simulink model "Excavator_Mevea_Bucket"  (R2026a)
settings: Solver=ode23t  StopTime=stopTime  FixedStep=1e-5  MaxStep=Ts  AbsTol=1e-3
PostLoadFcn:
  | set_param(bdroot,'IgnoredZcDiagnostic','none');
  | Excavator_Test_Scenario_Select('loadedBucketDigCycle');
  | Excavator_Mevea_params
StartFcn:
  | tStart = tic;
StopFcn:
  | elapsedSimTime = toc(tStart);
  | disp(['Elapsed Sim Time = ' num2str(elapsedSimTime)]);
model workspace: external: MAT-File ExcavatorAssemblyDataStruct.mat (data not in the file)
undefined symbols (not defined in the file or in its folder): AToBRegOrificeVector, AToTOrificeVector, BiPOrificeVector, BoomC, boomHEArea, boomREArea, boomUpMaxQ, boomValve, BToTOrificeVector, BucketC, bucketCloseMaxQ, bucketOpenMaxQ, BucketR, bucketValve, fluids, gravity, LeftBoomR, maxPumpDisp, minPumpDisp, nominalEngineSpeed, P28Assembly, PToAOrificeVector, PToBOrificeVector, pumpCmdNegRateLimit, pumpCmdPosRateLimit, RightBoomR, StickC, stickInMaxQ, stickOutMaxQ, StickR, stickValve, SwingC, swingDisplacement, swingHighSpeedThreshold, swingMaxQ, SwingR, swingSpeedQGain, swingValve, valveCmdNegRateLimit, valveCmdPosRateLimit, X, Y, Z
libraries: fl_lib x89, sm_lib x79, SimscapeFluids_lib x78, nesl_utility x57, simulink_extras x11, Excavator_Parts_Lib x6, SignalEditorBlockLib x1
(part 7 of 7)

== system Excavator_Mevea_Bucket/Excavator/Hydraulics/ValveBlocks/RightValveBlock/Boom Valve ==
  AtoBRegen : SimscapeFluids_lib/Isothermal Liquid/Valves & Orifices/Orifices/Orifice (IL)  orifice_type=foundation.enum.constant_variable.variable  constant_orifice_spec=fluids.isothermal_liquid.valves_orifices.orifices.enum.constant_orifice_spec.area  variable_orifice_spec=fluids.isothermal_liquid.valves_orifices.orifices.enum.orifice_spec.table1D_area_opening  orifice_area_constant=1e-3 m^2  p_diff_TLU_constant=[-4, -3, -2, -1, -.5, 0, .5, 1, 2, 3, 4] MPa  vol_flow_TLU_constant=[-2.44, -2.12, -1.68, -1.22, -.84, 0, .85, 1.21, 1.7, 2.09, 2.41] .* 1e-3 m^3/s  S_min=1e-10 m  del_S=0.005 m  open_orientation=fluids.isothermal_liquid.valves_orifices.orifices.enum.orifice_orientation.positive  area_max=0.5e-4 m^2  area_leak=1e-12 m^2  S_TLU=valveData.spoolPosVector mm  orifice_area_TLU=valveData.AtoBRegOrificeAreaVector mm^2  area=inf m^2  Cd=0.7  Re_c=150  smoothing_factor=0  pressure_recovery=simscape.enum.onoff.off  S_vol_flow_TLU=AToBRegOrificeVector - 1000*(0) mm  p_diff_TLU=[-10000000, -5000000, -2000000, 2000000, 5000000, 10000000] Pa  vol_flow_TLU=[-1e-07, -7.0711e-08, -4.4721e-08, 4.4721e-08, 7.0711e-08, 1e-07; -2.0352e-05, -1.4391e-05, -9.1017e-06, 9.1017e-06, 1.4391e-05, 2.0352e-05; -.0040736, -.0028805, -.0018218, .0018218, .0028805, .0040736; -.011438, -.0080879, -.0051152, .0051152, .0080879, .011438; -.034356, -.024293, -.015364, .015364, .024293, .034356] m^3/s
  AtoT : SimscapeFluids_lib/Isothermal Liquid/Valves & Orifices/Orifices/Orifice (IL)  orifice_type=foundation.enum.constant_variable.variable  constant_orifice_spec=fluids.isothermal_liquid.valves_orifices.orifices.enum.constant_orifice_spec.area  variable_orifice_spec=fluids.isothermal_liquid.valves_orifices.orifices.enum.orifice_spec.table1D_area_opening  orifice_area_constant=1e-3 m^2  p_diff_TLU_constant=[-4, -3, -2, -1, -.5, 0, .5, 1, 2, 3, 4] MPa  vol_flow_TLU_constant=[-2.44, -2.12, -1.68, -1.22, -.84, 0, .85, 1.21, 1.7, 2.09, 2.41] .* 1e-3 m^3/s  S_min=1e-10 m  del_S=0.005 m  open_orientation=fluids.isothermal_liquid.valves_orifices.orifices.enum.orifice_orientation.positive  area_max=0.5e-4 m^2  area_leak=1e-12 m^2  S_TLU=valveData.spoolPosVector mm  orifice_area_TLU=valveData.AtoTOrificeAreaVector mm^2  area=inf m^2  Cd=0.7  Re_c=150  smoothing_factor=0  pressure_recovery=simscape.enum.onoff.off  S_vol_flow_TLU=AToTOrificeVector - 1000*(0) mm  p_diff_TLU=[-10000000, -5000000, -2000000, 2000000, 5000000, 10000000] Pa  vol_flow_TLU=[-1e-07, -7.0711e-08, -4.4721e-08, 4.4721e-08, 7.0711e-08, 1e-07; -2.0352e-05, -1.4391e-05, -9.1017e-06, 9.1017e-06, 1.4391e-05, 2.0352e-05; -.0040736, -.0028805, -.0018218, .0018218, .0028805, .0040736; -.011438, -.0080879, -.0051152, .0051152, .0080879, .011438; -.034356, -.024293, -.015364, .015364, .024293, .034356] m^3/s
  BiPOrifice : SimscapeFluids_lib/Isothermal Liquid/Valves & Orifices/Orifices/Orifice (IL)  orifice_type=foundation.enum.constant_variable.variable  constant_orifice_spec=fluids.isothermal_liquid.valves_orifices.orifices.enum.constant_orifice_spec.area  variable_orifice_spec=fluids.isothermal_liquid.valves_orifices.orifices.enum.orifice_spec.table1D_area_opening  orifice_area_constant=1e-3 m^2  p_diff_TLU_constant=[-4, -3, -2, -1, -.5, 0, .5, 1, 2, 3, 4] MPa  vol_flow_TLU_constant=[-2.44, -2.12, -1.68, -1.22, -.84, 0, .85, 1.21, 1.7, 2.09, 2.41] .* 1e-3 m^3/s  S_min=1e-10 m  del_S=0.005 m  open_orientation=fluids.isothermal_liquid.valves_orifices.orifices.enum.orifice_orientation.positive  area_max=0.5e-4 m^2  area_leak=1e-12 m^2  S_TLU=valveData.spoolPosVector mm  orifice_area_TLU=valveData.BiPOrificeAreaVector mm^2  area=inf m^2  Cd=0.7  Re_c=150  smoothing_factor=0  pressure_recovery=simscape.enum.onoff.off  S_vol_flow_TLU=BiPOrificeVector - 1000*(0) mm  p_diff_TLU=[-10000000, -5000000, -2000000, 2000000, 5000000, 10000000] Pa  vol_flow_TLU=[-1e-07, -7.0711e-08, -4.4721e-08, 4.4721e-08, 7.0711e-08, 1e-07; -2.0352e-05, -1.4391e-05, -9.1017e-06, 9.1017e-06, 1.4391e-05, 2.0352e-05; -.0040736, -.0028805, -.0018218, .0018218, .0028805, .0040736; -.011438, -.0080879, -.0051152, .0051152, .0080879, .011438; -.034356, -.024293, -.015364, .015364, .024293, .034356] m^3/s
  BoomRegenCV : SimscapeFluids_lib/Isothermal Liquid/Valves & Orifices/Directional Control Valves/Check Valve (IL)  opening_spec=2*(fluids.isothermal_liquid.valves_orifices.enum.opening_spec.linear)-1  pressure_control_spec=fluids.isothermal_liquid.valves_orifices.enum.pressure_control_spec.dp  p_crack_differential=valveData.checkValveCrackingPrDiff bar  p_crack_gauge=0.1 MPa  press_max_differential=valveData.checkValveMaxOpeningPrDiff bar  press_max_gauge=0.2 MPa  area_max=valveData.checkValveMaxOpeningArea mm^2  area_leak=valveData.checkValveLeakageArea mm^2  p_diff_TLU=[0.01 : 0.01 : 0.1] MPa  valve_area_TLU=[1e-10, 1e-05, 2e-05, 3e-05, 4e-05, 5e-05, 6e-05, 7.5e-05, 8.5e-05, .0001] m^2  vol_flow_TLU=[.000358, .045, .11, .191, .284, .39, .505, .63, .764, .905] .* 1e-3 m^3/s  area=inf m^2  Cd=0.7  Re_c=150  smoothing_factor=0.1  pressure_recovery=simscape.enum.onoff.off  opening_dynamics=simscape.enum.onoff.off  tau=0.1 s
  BtoT : SimscapeFluids_lib/Isothermal Liquid/Valves & Orifices/Orifices/Orifice (IL)  orifice_type=foundation.enum.constant_variable.variable  constant_orifice_spec=fluids.isothermal_liquid.valves_orifices.orifices.enum.constant_orifice_spec.area  variable_orifice_spec=fluids.isothermal_liquid.valves_orifices.orifices.enum.orifice_spec.table1D_area_opening  orifice_area_constant=1e-3 m^2  p_diff_TLU_constant=[-4, -3, -2, -1, -.5, 0, .5, 1, 2, 3, 4] MPa  vol_flow_TLU_constant=[-2.44, -2.12, -1.68, -1.22, -.84, 0, .85, 1.21, 1.7, 2.09, 2.41] .* 1e-3 m^3/s  S_min=1e-10 m  del_S=0.005 m  open_orientation=fluids.isothermal_liquid.valves_orifices.orifices.enum.orifice_orientation.positive  area_max=0.5e-4 m^2  area_leak=1e-12 m^2  S_TLU=valveData.spoolPosVector mm  orifice_area_TLU=valveData.BtoTOrificeAreaVector mm^2  area=inf m^2  Cd=0.7  Re_c=150  smoothing_factor=0  pressure_recovery=simscape.enum.onoff.off  S_vol_flow_TLU=BToTOrificeVector - 1000*(0) mm  p_diff_TLU=[-10000000, -5000000, -2000000, 2000000, 5000000, 10000000] Pa  vol_flow_TLU=[-1e-07, -7.0711e-08, -4.4721e-08, 4.4721e-08, 7.0711e-08, 1e-07; -2.0352e-05, -1.4391e-05, -9.1017e-06, 9.1017e-06, 1.4391e-05, 2.0352e-05; -.0040736, -.0028805, -.0018218, .0018218, .0028805, .0040736; -.011438, -.0080879, -.0051152, .0051152, .0080879, .011438; -.034356, -.024293, -.015364, .015364, .024293, .034356] m^3/s
  PS Abs : fl_lib/Physical Signals/Nonlinear Operators/PS Abs  ZeroCross=true
  PS Gain1 : fl_lib/Physical Signals/Functions/PS Gain  gain=-1
  PtoA : SimscapeFluids_lib/Isothermal Liquid/Valves & Orifices/Orifices/Orifice (IL)  orifice_type=foundation.enum.constant_variable.variable  constant_orifice_spec=fluids.isothermal_liquid.valves_orifices.orifices.enum.constant_orifice_spec.area  variable_orifice_spec=fluids.isothermal_liquid.valves_orifices.orifices.enum.orifice_spec.table1D_area_opening  orifice_area_constant=1e-3 m^2  p_diff_TLU_constant=[-4, -3, -2, -1, -.5, 0, .5, 1, 2, 3, 4] MPa  vol_flow_TLU_constant=[-2.44, -2.12, -1.68, -1.22, -.84, 0, .85, 1.21, 1.7, 2.09, 2.41] .* 1e-3 m^3/s  S_min=1e-10 m  del_S=0.005 m  open_orientation=fluids.isothermal_liquid.valves_orifices.orifices.enum.orifice_orientation.positive  area_max=0.5e-4 m^2  area_leak=1e-12 m^2  S_TLU=valveData.spoolPosVector mm  orifice_area_TLU=valveData.PtoAOrificeAreaVector mm^2  area=inf m^2  Cd=0.7  Re_c=150  smoothing_factor=0  pressure_recovery=simscape.enum.onoff.off  S_vol_flow_TLU=PToAOrificeVector - 1000*(0) mm  p_diff_TLU=[-10000000, -5000000, -2000000, 2000000, 5000000, 10000000] Pa  vol_flow_TLU=[-1e-07, -7.0711e-08, -4.4721e-08, 4.4721e-08, 7.0711e-08, 1e-07; -2.0352e-05, -1.4391e-05, -9.1017e-06, 9.1017e-06, 1.4391e-05, 2.0352e-05; -.0040736, -.0028805, -.0018218, .0018218, .0028805, .0040736; -.011438, -.0080879, -.0051152, .0051152, .0080879, .011438; -.034356, -.024293, -.015364, .015364, .024293, .034356] m^3/s
  PtoB : SimscapeFluids_lib/Isothermal Liquid/Valves & Orifices/Orifices/Orifice (IL)  orifice_type=foundation.enum.constant_variable.variable  constant_orifice_spec=fluids.isothermal_liquid.valves_orifices.orifices.enum.constant_orifice_spec.area  variable_orifice_spec=fluids.isothermal_liquid.valves_orifices.orifices.enum.orifice_spec.table1D_area_opening  orifice_area_constant=1e-3 m^2  p_diff_TLU_constant=[-4, -3, -2, -1, -.5, 0, .5, 1, 2, 3, 4] MPa  vol_flow_TLU_constant=[-2.44, -2.12, -1.68, -1.22, -.84, 0, .85, 1.21, 1.7, 2.09, 2.41] .* 1e-3 m^3/s  S_min=1e-10 m  del_S=0.005 m  open_orientation=fluids.isothermal_liquid.valves_orifices.orifices.enum.orifice_orientation.positive  area_max=0.5e-4 m^2  area_leak=1e-12 m^2  S_TLU=valveData.spoolPosVector mm  orifice_area_TLU=valveData.PtoBOrificeAreaVector mm^2  area=inf m^2  Cd=0.7  Re_c=150  smoothing_factor=0  pressure_recovery=simscape.enum.onoff.off  S_vol_flow_TLU=PToBOrificeVector - 1000*(0) mm  p_diff_TLU=[-10000000, -5000000, -2000000, 2000000, 5000000, 10000000] Pa  vol_flow_TLU=[-1e-07, -7.0711e-08, -4.4721e-08, 4.4721e-08, 7.0711e-08, 1e-07; -2.0352e-05, -1.4391e-05, -9.1017e-06, 9.1017e-06, 1.4391e-05, 2.0352e-05; -.0040736, -.0028805, -.0018218, .0018218, .0028805, .0040736; -.011438, -.0080879, -.0051152, .0051152, .0080879, .011438; -.034356, -.024293, -.015364, .015364, .024293, .034356] m^3/s
  Volume Regen Valve : fl_lib/Isothermal Liquid/Elements/Constant Volume Chamber (IL)  volume=vcVol m^3  p_I_specify=on  p_I_priority=High  p_I=initBoomREPr bar  p_I_nominal_specify=off  p_I_nominal_value=1  p_I_nominal_unit=MPa
  S : PMIOPort  Side=Left
  P : PMIOPort  Port=2  Side=Left
  T : PMIOPort  Port=3  Side=Left
  BiPIn : PMIOPort  Port=4  Side=Left
  A : PMIOPort  Port=5  Side=Right
  B : PMIOPort  Port=6  Side=Right
  BiPOut : PMIOPort  Port=7  Side=Right
  connections:
  BtoT/LConn2 -- PS Gain1/RConn1 -- PtoA/LConn2
  PS Abs/LConn1 -- S/RConn1 -- AtoT/LConn2 -- AtoBRegen/LConn2 -- PtoB/LConn2 -- PS Gain1/LConn1
  AtoBRegen/RConn1 -- Volume Regen Valve/LConn1 -- BoomRegenCV/LConn1
  BtoT/RConn1 -- AtoT/RConn1 -- T/RConn1
  BiPOrifice/RConn1 -- BiPOut/RConn1
  BiPOrifice/LConn1 -- BiPIn/RConn1
  AtoBRegen/LConn1 -- A/RConn1 -- AtoT/LConn1 -- PtoA/RConn1
  PtoA/LConn1 -- PtoB/LConn1 -- P/RConn1
  BtoT/LConn1 -- B/RConn1 -- BoomRegenCV/RConn1 -- PtoB/RConn1
  PS Abs/RConn1 -- BiPOrifice/LConn2

== system Excavator_Mevea_Bucket/Excavator/Hydraulics/ValveBlocks/RightValveBlock/Bucket Valve ==
  AtoT : SimscapeFluids_lib/Isothermal Liquid/Valves & Orifices/Orifices/Orifice (IL)  orifice_type=foundation.enum.constant_variable.variable  constant_orifice_spec=fluids.isothermal_liquid.valves_orifices.orifices.enum.constant_orifice_spec.area  variable_orifice_spec=fluids.isothermal_liquid.valves_orifices.orifices.enum.orifice_spec.table1D_area_opening  orifice_area_constant=1e-3 m^2  p_diff_TLU_constant=[-4, -3, -2, -1, -.5, 0, .5, 1, 2, 3, 4] MPa  vol_flow_TLU_constant=[-2.44, -2.12, -1.68, -1.22, -.84, 0, .85, 1.21, 1.7, 2.09, 2.41] .* 1e-3 m^3/s  S_min=1e-10 m  del_S=0.005 m  open_orientation=fluids.isothermal_liquid.valves_orifices.orifices.enum.orifice_orientation.positive  area_max=0.5e-4 m^2  area_leak=1e-12 m^2  S_TLU=valveData.spoolPosVector mm  orifice_area_TLU=valveData.AtoTOrificeAreaVector mm^2  area=inf m^2  Cd=0.7  Re_c=150  smoothing_factor=0  pressure_recovery=simscape.enum.onoff.off  S_vol_flow_TLU=AToTOrificeVector - 1000*(0) mm  p_diff_TLU=[-10000000, -5000000, -2000000, 2000000, 5000000, 10000000] Pa  vol_flow_TLU=[-1e-07, -7.0711e-08, -4.4721e-08, 4.4721e-08, 7.0711e-08, 1e-07; -2.0352e-05, -1.4391e-05, -9.1017e-06, 9.1017e-06, 1.4391e-05, 2.0352e-05; -.0040736, -.0028805, -.0018218, .0018218, .0028805, .0040736; -.011438, -.0080879, -.0051152, .0051152, .0080879, .011438; -.034356, -.024293, -.015364, .015364, .024293, .034356] m^3/s
  BiPOrifice : SimscapeFluids_lib/Isothermal Liquid/Valves & Orifices/Orifices/Orifice (IL)  orifice_type=foundation.enum.constant_variable.variable  constant_orifice_spec=fluids.isothermal_liquid.valves_orifices.orifices.enum.constant_orifice_spec.area  variable_orifice_spec=fluids.isothermal_liquid.valves_orifices.orifices.enum.orifice_spec.table1D_area_opening  orifice_area_constant=1e-3 m^2  p_diff_TLU_constant=[-4, -3, -2, -1, -.5, 0, .5, 1, 2, 3, 4] MPa  vol_flow_TLU_constant=[-2.44, -2.12, -1.68, -1.22, -.84, 0, .85, 1.21, 1.7, 2.09, 2.41] .* 1e-3 m^3/s  S_min=1e-10 m  del_S=0.005 m  open_orientation=fluids.isothermal_liquid.valves_orifices.orifices.enum.orifice_orientation.positive  area_max=0.5e-4 m^2  area_leak=1e-12 m^2  S_TLU=valveData.spoolPosVector mm  orifice_area_TLU=valveData.BiPOrificeAreaVector mm^2  area=inf m^2  Cd=0.7  Re_c=150  smoothing_factor=0  pressure_recovery=simscape.enum.onoff.off  S_vol_flow_TLU=BiPOrificeVector - 1000*(0) mm  p_diff_TLU=[-10000000, -5000000, -2000000, 2000000, 5000000, 10000000] Pa  vol_flow_TLU=[-1e-07, -7.0711e-08, -4.4721e-08, 4.4721e-08, 7.0711e-08, 1e-07; -2.0352e-05, -1.4391e-05, -9.1017e-06, 9.1017e-06, 1.4391e-05, 2.0352e-05; -.0040736, -.0028805, -.0018218, .0018218, .0028805, .0040736; -.011438, -.0080879, -.0051152, .0051152, .0080879, .011438; -.034356, -.024293, -.015364, .015364, .024293, .034356] m^3/s
  BtoT : SimscapeFluids_lib/Isothermal Liquid/Valves & Orifices/Orifices/Orifice (IL)  orifice_type=foundation.enum.constant_variable.variable  constant_orifice_spec=fluids.isothermal_liquid.valves_orifices.orifices.enum.constant_orifice_spec.area  variable_orifice_spec=fluids.isothermal_liquid.valves_orifices.orifices.enum.orifice_spec.table1D_area_opening  orifice_area_constant=1e-3 m^2  p_diff_TLU_constant=[-4, -3, -2, -1, -.5, 0, .5, 1, 2, 3, 4] MPa  vol_flow_TLU_constant=[-2.44, -2.12, -1.68, -1.22, -.84, 0, .85, 1.21, 1.7, 2.09, 2.41] .* 1e-3 m^3/s  S_min=1e-10 m  del_S=0.005 m  open_orientation=fluids.isothermal_liquid.valves_orifices.orifices.enum.orifice_orientation.positive  area_max=0.5e-4 m^2  area_leak=1e-12 m^2  S_TLU=valveData.spoolPosVector mm  orifice_area_TLU=valveData.BtoTOrificeAreaVector mm^2  area=inf m^2  Cd=0.7  Re_c=150  smoothing_factor=0  pressure_recovery=simscape.enum.onoff.off  S_vol_flow_TLU=BToTOrificeVector - 1000*(0) mm  p_diff_TLU=[-10000000, -5000000, -2000000, 2000000, 5000000, 10000000] Pa  vol_flow_TLU=[-1e-07, -7.0711e-08, -4.4721e-08, 4.4721e-08, 7.0711e-08, 1e-07; -2.0352e-05, -1.4391e-05, -9.1017e-06, 9.1017e-06, 1.4391e-05, 2.0352e-05; -.0040736, -.0028805, -.0018218, .0018218, .0028805, .0040736; -.011438, -.0080879, -.0051152, .0051152, .0080879, .011438; -.034356, -.024293, -.015364, .015364, .024293, .034356] m^3/s
  PS Abs : fl_lib/Physical Signals/Nonlinear Operators/PS Abs  ZeroCross=true
  PS Gain1 : fl_lib/Physical Signals/Functions/PS Gain  gain=-1
  PtoA : SimscapeFluids_lib/Isothermal Liquid/Valves & Orifices/Orifices/Orifice (IL)  orifice_type=foundation.enum.constant_variable.variable  constant_orifice_spec=fluids.isothermal_liquid.valves_orifices.orifices.enum.constant_orifice_spec.area  variable_orifice_spec=fluids.isothermal_liquid.valves_orifices.orifices.enum.orifice_spec.table1D_area_opening  orifice_area_constant=1e-3 m^2  p_diff_TLU_constant=[-4, -3, -2, -1, -.5, 0, .5, 1, 2, 3, 4] MPa  vol_flow_TLU_constant=[-2.44, -2.12, -1.68, -1.22, -.84, 0, .85, 1.21, 1.7, 2.09, 2.41] .* 1e-3 m^3/s  S_min=1e-10 m  del_S=0.005 m  open_orientation=fluids.isothermal_liquid.valves_orifices.orifices.enum.orifice_orientation.positive  area_max=0.5e-4 m^2  area_leak=1e-12 m^2  S_TLU=valveData.spoolPosVector mm  orifice_area_TLU=valveData.PtoAOrificeAreaVector mm^2  area=inf m^2  Cd=0.7  Re_c=150  smoothing_factor=0  pressure_recovery=simscape.enum.onoff.off  S_vol_flow_TLU=PToAOrificeVector - 1000*(0) mm  p_diff_TLU=[-10000000, -5000000, -2000000, 2000000, 5000000, 10000000] Pa  vol_flow_TLU=[-1e-07, -7.0711e-08, -4.4721e-08, 4.4721e-08, 7.0711e-08, 1e-07; -2.0352e-05, -1.4391e-05, -9.1017e-06, 9.1017e-06, 1.4391e-05, 2.0352e-05; -.0040736, -.0028805, -.0018218, .0018218, .0028805, .0040736; -.011438, -.0080879, -.0051152, .0051152, .0080879, .011438; -.034356, -.024293, -.015364, .015364, .024293, .034356] m^3/s
  PtoB : SimscapeFluids_lib/Isothermal Liquid/Valves & Orifices/Orifices/Orifice (IL)  orifice_type=foundation.enum.constant_variable.variable  constant_orifice_spec=fluids.isothermal_liquid.valves_orifices.orifices.enum.constant_orifice_spec.area  variable_orifice_spec=fluids.isothermal_liquid.valves_orifices.orifices.enum.orifice_spec.table1D_area_opening  orifice_area_constant=1e-3 m^2  p_diff_TLU_constant=[-4, -3, -2, -1, -.5, 0, .5, 1, 2, 3, 4] MPa  vol_flow_TLU_constant=[-2.44, -2.12, -1.68, -1.22, -.84, 0, .85, 1.21, 1.7, 2.09, 2.41] .* 1e-3 m^3/s  S_min=1e-10 m  del_S=0.005 m  open_orientation=fluids.isothermal_liquid.valves_orifices.orifices.enum.orifice_orientation.positive  area_max=0.5e-4 m^2  area_leak=1e-12 m^2  S_TLU=valveData.spoolPosVector mm  orifice_area_TLU=valveData.PtoBOrificeAreaVector mm^2  area=inf m^2  Cd=0.7  Re_c=150  smoothing_factor=0  pressure_recovery=simscape.enum.onoff.off  S_vol_flow_TLU=PToBOrificeVector - 1000*(0) mm  p_diff_TLU=[-10000000, -5000000, -2000000, 2000000, 5000000, 10000000] Pa  vol_flow_TLU=[-1e-07, -7.0711e-08, -4.4721e-08, 4.4721e-08, 7.0711e-08, 1e-07; -2.0352e-05, -1.4391e-05, -9.1017e-06, 9.1017e-06, 1.4391e-05, 2.0352e-05; -.0040736, -.0028805, -.0018218, .0018218, .0028805, .0040736; -.011438, -.0080879, -.0051152, .0051152, .0080879, .011438; -.034356, -.024293, -.015364, .015364, .024293, .034356] m^3/s
  S : PMIOPort  Side=Left
  P : PMIOPort  Port=2  Side=Left
  T : PMIOPort  Port=3  Side=Left
  BiPIn : PMIOPort  Port=4  Side=Left
  A : PMIOPort  Port=5  Side=Right
  B : PMIOPort  Port=6  Side=Right
  BiPOut : PMIOPort  Port=7  Side=Right
  connections:
  BtoT/LConn2 -- PtoA/LConn2 -- PS Gain1/RConn1
  BiPOrifice/LConn2 -- PS Abs/RConn1
  S/RConn1 -- PtoB/LConn2 -- AtoT/LConn2 -- PS Gain1/LConn1 -- PS Abs/LConn1
  T/RConn1 -- BtoT/RConn1 -- AtoT/RConn1
  BiPOrifice/RConn1 -- BiPOut/RConn1
  BiPOrifice/LConn1 -- BiPIn/RConn1
  PtoA/RConn1 -- A/RConn1 -- AtoT/LConn1
  PtoB/LConn1 -- P/RConn1 -- PtoA/LConn1
  PtoB/RConn1 -- BtoT/LConn1 -- B/RConn1

== system Excavator_Mevea_Bucket/Excavator/Hydraulics/ValveBlocks/RightValveBlock/Cmd to Spool Pos ==
  Cmds : Inport
  Bus Selector : BusSelector  OutputSignals=BMSpoolPos,SKSpoolPos,BTSpoolPos
  Simulink-PS Converter : nesl_utility/Simulink-PS Converter  PhysicalDomain=network_engine_domain  SubClassName=ps_input  LeftPortType=input  RightPortType=output  PseudoPeriodic=off  Frequencies=[]  NoiseDistribution=none  NoiseParameters=[]  Unit=mm  AffineConversion=off  FilteringAndDerivatives=provide  SimscapeFilterOrder=1  InputFilterTimeConstant=0.01  UdotUserProvided=0
  Simulink-PS Converter1 : nesl_utility/Simulink-PS Converter  PhysicalDomain=network_engine_domain  SubClassName=ps_input  LeftPortType=input  RightPortType=output  PseudoPeriodic=off  Frequencies=[]  NoiseDistribution=none  NoiseParameters=[]  Unit=mm  AffineConversion=off  FilteringAndDerivatives=provide  SimscapeFilterOrder=1  InputFilterTimeConstant=0.01  UdotUserProvided=0
  Simulink-PS Converter2 : nesl_utility/Simulink-PS Converter  PhysicalDomain=network_engine_domain  SubClassName=ps_input  LeftPortType=input  RightPortType=output  PseudoPeriodic=off  Frequencies=[]  NoiseDistribution=none  NoiseParameters=[]  Unit=mm  AffineConversion=off  FilteringAndDerivatives=provide  SimscapeFilterOrder=1  InputFilterTimeConstant=0.01  UdotUserProvided=0
  BMPos : PMIOPort  Side=Right
  SKPos : PMIOPort  Port=2  Side=Right
  BTPos : PMIOPort  Port=3  Side=Right
  wires:
  Bus Selector/1 -> Simulink-PS Converter/1  "<BMSpoolPos>"
  Bus Selector/3 -> Simulink-PS Converter2/1  "<BTSpoolPos>"
  Bus Selector/2 -> Simulink-PS Converter1/1  "<SKSpoolPos>"
  Cmds/1 -> Bus Selector/1
  connections:
  Simulink-PS Converter/RConn1 -- BMPos/RConn1
  Simulink-PS Converter1/RConn1 -- SKPos/RConn1
  Simulink-PS Converter2/RConn1 -- BTPos/RConn1

== system Excavator_Mevea_Bucket/Excavator/Hydraulics/ValveBlocks/RightValveBlock/Stick Valve ==
  AtoT : SimscapeFluids_lib/Isothermal Liquid/Valves & Orifices/Orifices/Orifice (IL)  orifice_type=foundation.enum.constant_variable.variable  constant_orifice_spec=fluids.isothermal_liquid.valves_orifices.orifices.enum.constant_orifice_spec.area  variable_orifice_spec=fluids.isothermal_liquid.valves_orifices.orifices.enum.orifice_spec.table1D_area_opening  orifice_area_constant=1e-3 m^2  p_diff_TLU_constant=[-4, -3, -2, -1, -.5, 0, .5, 1, 2, 3, 4] MPa  vol_flow_TLU_constant=[-2.44, -2.12, -1.68, -1.22, -.84, 0, .85, 1.21, 1.7, 2.09, 2.41] .* 1e-3 m^3/s  S_min=1e-10 m  del_S=0.005 m  open_orientation=fluids.isothermal_liquid.valves_orifices.orifices.enum.orifice_orientation.positive  area_max=0.5e-4 m^2  area_leak=1e-12 m^2  S_TLU=valveData.spoolPosVector mm  orifice_area_TLU=valveData.AtoTOrificeAreaVector mm^2  area=inf m^2  Cd=0.7  Re_c=150  smoothing_factor=0  pressure_recovery=simscape.enum.onoff.off  S_vol_flow_TLU=AToTOrificeVector - 1000*(0) mm  p_diff_TLU=[-10000000, -5000000, -2000000, 2000000, 5000000, 10000000] Pa  vol_flow_TLU=[-1e-07, -7.0711e-08, -4.4721e-08, 4.4721e-08, 7.0711e-08, 1e-07; -2.0352e-05, -1.4391e-05, -9.1017e-06, 9.1017e-06, 1.4391e-05, 2.0352e-05; -.0040736, -.0028805, -.0018218, .0018218, .0028805, .0040736; -.011438, -.0080879, -.0051152, .0051152, .0080879, .011438; -.034356, -.024293, -.015364, .015364, .024293, .034356] m^3/s
  BiPOrifice : SimscapeFluids_lib/Isothermal Liquid/Valves & Orifices/Orifices/Orifice (IL)  orifice_type=foundation.enum.constant_variable.variable  constant_orifice_spec=fluids.isothermal_liquid.valves_orifices.orifices.enum.constant_orifice_spec.area  variable_orifice_spec=fluids.isothermal_liquid.valves_orifices.orifices.enum.orifice_spec.table1D_area_opening  orifice_area_constant=1e-3 m^2  p_diff_TLU_constant=[-4, -3, -2, -1, -.5, 0, .5, 1, 2, 3, 4] MPa  vol_flow_TLU_constant=[-2.44, -2.12, -1.68, -1.22, -.84, 0, .85, 1.21, 1.7, 2.09, 2.41] .* 1e-3 m^3/s  S_min=1e-10 m  del_S=0.005 m  open_orientation=fluids.isothermal_liquid.valves_orifices.orifices.enum.orifice_orientation.positive  area_max=0.5e-4 m^2  area_leak=1e-12 m^2  S_TLU=valveData.spoolPosVector mm  orifice_area_TLU=valveData.BiPOrificeAreaVector mm^2  area=inf m^2  Cd=0.7  Re_c=150  smoothing_factor=0  pressure_recovery=simscape.enum.onoff.off  S_vol_flow_TLU=BiPOrificeVector - 1000*(0) mm  p_diff_TLU=[-10000000, -5000000, -2000000, 2000000, 5000000, 10000000] Pa  vol_flow_TLU=[-1e-07, -7.0711e-08, -4.4721e-08, 4.4721e-08, 7.0711e-08, 1e-07; -2.0352e-05, -1.4391e-05, -9.1017e-06, 9.1017e-06, 1.4391e-05, 2.0352e-05; -.0040736, -.0028805, -.0018218, .0018218, .0028805, .0040736; -.011438, -.0080879, -.0051152, .0051152, .0080879, .011438; -.034356, -.024293, -.015364, .015364, .024293, .034356] m^3/s
  BtoARegen : SimscapeFluids_lib/Isothermal Liquid/Valves & Orifices/Orifices/Orifice (IL)  orifice_type=foundation.enum.constant_variable.variable  constant_orifice_spec=fluids.isothermal_liquid.valves_orifices.orifices.enum.constant_orifice_spec.area  variable_orifice_spec=fluids.isothermal_liquid.valves_orifices.orifices.enum.orifice_spec.table1D_area_opening  orifice_area_constant=1e-3 m^2  p_diff_TLU_constant=[-4, -3, -2, -1, -.5, 0, .5, 1, 2, 3, 4] MPa  vol_flow_TLU_constant=[-2.44, -2.12, -1.68, -1.22, -.84, 0, .85, 1.21, 1.7, 2.09, 2.41] .* 1e-3 m^3/s  S_min=1e-10 m  del_S=0.005 m  open_orientation=fluids.isothermal_liquid.valves_orifices.orifices.enum.orifice_orientation.positive  area_max=0.5e-4 m^2  area_leak=1e-12 m^2  S_TLU=valveData.spoolPosVector mm  orifice_area_TLU=valveData.BtoARegOrificeAreaVector mm^2  area=inf m^2  Cd=0.7  Re_c=150  smoothing_factor=0  pressure_recovery=simscape.enum.onoff.off  S_vol_flow_TLU=AToBRegOrificeVector - 1000*(0) mm  p_diff_TLU=[-10000000, -5000000, -2000000, 2000000, 5000000, 10000000] Pa  vol_flow_TLU=[-1e-07, -7.0711e-08, -4.4721e-08, 4.4721e-08, 7.0711e-08, 1e-07; -2.0352e-05, -1.4391e-05, -9.1017e-06, 9.1017e-06, 1.4391e-05, 2.0352e-05; -.0040736, -.0028805, -.0018218, .0018218, .0028805, .0040736; -.011438, -.0080879, -.0051152, .0051152, .0080879, .011438; -.034356, -.024293, -.015364, .015364, .024293, .034356] m^3/s
  BtoT : SimscapeFluids_lib/Isothermal Liquid/Valves & Orifices/Orifices/Orifice (IL)  orifice_type=foundation.enum.constant_variable.variable  constant_orifice_spec=fluids.isothermal_liquid.valves_orifices.orifices.enum.constant_orifice_spec.area  variable_orifice_spec=fluids.isothermal_liquid.valves_orifices.orifices.enum.orifice_spec.table1D_area_opening  orifice_area_constant=1e-3 m^2  p_diff_TLU_constant=[-4, -3, -2, -1, -.5, 0, .5, 1, 2, 3, 4] MPa  vol_flow_TLU_constant=[-2.44, -2.12, -1.68, -1.22, -.84, 0, .85, 1.21, 1.7, 2.09, 2.41] .* 1e-3 m^3/s  S_min=1e-10 m  del_S=0.005 m  open_orientation=fluids.isothermal_liquid.valves_orifices.orifices.enum.orifice_orientation.positive  area_max=0.5e-4 m^2  area_leak=1e-12 m^2  S_TLU=valveData.spoolPosVector mm  orifice_area_TLU=valveData.BtoTOrificeAreaVector mm^2  area=inf m^2  Cd=0.7  Re_c=150  smoothing_factor=0  pressure_recovery=simscape.enum.onoff.off  S_vol_flow_TLU=BToTOrificeVector - 1000*(0) mm  p_diff_TLU=[-10000000, -5000000, -2000000, 2000000, 5000000, 10000000] Pa  vol_flow_TLU=[-1e-07, -7.0711e-08, -4.4721e-08, 4.4721e-08, 7.0711e-08, 1e-07; -2.0352e-05, -1.4391e-05, -9.1017e-06, 9.1017e-06, 1.4391e-05, 2.0352e-05; -.0040736, -.0028805, -.0018218, .0018218, .0028805, .0040736; -.011438, -.0080879, -.0051152, .0051152, .0080879, .011438; -.034356, -.024293, -.015364, .015364, .024293, .034356] m^3/s
  PS Abs : fl_lib/Physical Signals/Nonlinear Operators/PS Abs  ZeroCross=true
  PS Gain1 : fl_lib/Physical Signals/Functions/PS Gain  gain=-1
  PtoA : SimscapeFluids_lib/Isothermal Liquid/Valves & Orifices/Orifices/Orifice (IL)  orifice_type=foundation.enum.constant_variable.variable  constant_orifice_spec=fluids.isothermal_liquid.valves_orifices.orifices.enum.constant_orifice_spec.area  variable_orifice_spec=fluids.isothermal_liquid.valves_orifices.orifices.enum.orifice_spec.table1D_area_opening  orifice_area_constant=1e-3 m^2  p_diff_TLU_constant=[-4, -3, -2, -1, -.5, 0, .5, 1, 2, 3, 4] MPa  vol_flow_TLU_constant=[-2.44, -2.12, -1.68, -1.22, -.84, 0, .85, 1.21, 1.7, 2.09, 2.41] .* 1e-3 m^3/s  S_min=1e-10 m  del_S=0.005 m  open_orientation=fluids.isothermal_liquid.valves_orifices.orifices.enum.orifice_orientation.positive  area_max=0.5e-4 m^2  area_leak=1e-12 m^2  S_TLU=valveData.spoolPosVector mm  orifice_area_TLU=valveData.PtoAOrificeAreaVector mm^2  area=inf m^2  Cd=0.7  Re_c=150  smoothing_factor=0  pressure_recovery=simscape.enum.onoff.off  S_vol_flow_TLU=PToAOrificeVector - 1000*(0) mm  p_diff_TLU=[-10000000, -5000000, -2000000, 2000000, 5000000, 10000000] Pa  vol_flow_TLU=[-1e-07, -7.0711e-08, -4.4721e-08, 4.4721e-08, 7.0711e-08, 1e-07; -2.0352e-05, -1.4391e-05, -9.1017e-06, 9.1017e-06, 1.4391e-05, 2.0352e-05; -.0040736, -.0028805, -.0018218, .0018218, .0028805, .0040736; -.011438, -.0080879, -.0051152, .0051152, .0080879, .011438; -.034356, -.024293, -.015364, .015364, .024293, .034356] m^3/s
  PtoB : SimscapeFluids_lib/Isothermal Liquid/Valves & Orifices/Orifices/Orifice (IL)  orifice_type=foundation.enum.constant_variable.variable  constant_orifice_spec=fluids.isothermal_liquid.valves_orifices.orifices.enum.constant_orifice_spec.area  variable_orifice_spec=fluids.isothermal_liquid.valves_orifices.orifices.enum.orifice_spec.table1D_area_opening  orifice_area_constant=1e-3 m^2  p_diff_TLU_constant=[-4, -3, -2, -1, -.5, 0, .5, 1, 2, 3, 4] MPa  vol_flow_TLU_constant=[-2.44, -2.12, -1.68, -1.22, -.84, 0, .85, 1.21, 1.7, 2.09, 2.41] .* 1e-3 m^3/s  S_min=1e-10 m  del_S=0.005 m  open_orientation=fluids.isothermal_liquid.valves_orifices.orifices.enum.orifice_orientation.positive  area_max=0.5e-4 m^2  area_leak=1e-12 m^2  S_TLU=valveData.spoolPosVector mm  orifice_area_TLU=valveData.PtoBOrificeAreaVector mm^2  area=inf m^2  Cd=0.7  Re_c=150  smoothing_factor=0  pressure_recovery=simscape.enum.onoff.off  S_vol_flow_TLU=PToBOrificeVector - 1000*(0) mm  p_diff_TLU=[-10000000, -5000000, -2000000, 2000000, 5000000, 10000000] Pa  vol_flow_TLU=[-1e-07, -7.0711e-08, -4.4721e-08, 4.4721e-08, 7.0711e-08, 1e-07; -2.0352e-05, -1.4391e-05, -9.1017e-06, 9.1017e-06, 1.4391e-05, 2.0352e-05; -.0040736, -.0028805, -.0018218, .0018218, .0028805, .0040736; -.011438, -.0080879, -.0051152, .0051152, .0080879, .011438; -.034356, -.024293, -.015364, .015364, .024293, .034356] m^3/s
  StickRegenCV : SimscapeFluids_lib/Isothermal Liquid/Valves & Orifices/Directional Control Valves/Check Valve (IL)  opening_spec=2*(fluids.isothermal_liquid.valves_orifices.enum.opening_spec.linear)-1  pressure_control_spec=fluids.isothermal_liquid.valves_orifices.enum.pressure_control_spec.dp  p_crack_differential=valveData.checkValveCrackingPrDiff bar  p_crack_gauge=0.1 MPa  press_max_differential=valveData.checkValveMaxOpeningPrDiff bar  press_max_gauge=0.2 MPa  area_max=valveData.checkValveMaxOpeningArea mm^2  area_leak=valveData.checkValveLeakageArea mm^2  p_diff_TLU=[0.01 : 0.01 : 0.1] MPa  valve_area_TLU=[1e-10, 1e-05, 2e-05, 3e-05, 4e-05, 5e-05, 6e-05, 7.5e-05, 8.5e-05, .0001] m^2  vol_flow_TLU=[.000358, .045, .11, .191, .284, .39, .505, .63, .764, .905] .* 1e-3 m^3/s  area=inf m^2  Cd=0.7  Re_c=150  smoothing_factor=0.1  pressure_recovery=simscape.enum.onoff.off  opening_dynamics=simscape.enum.onoff.off  tau=0.1 s
  Volume Regen Valve : fl_lib/Isothermal Liquid/Elements/Constant Volume Chamber (IL)  volume=vcVol m^3  p_I_specify=on  p_I_priority=High  p_I=initStickHEPr bar  p_I_nominal_specify=off  p_I_nominal_value=1  p_I_nominal_unit=MPa
  S : PMIOPort  Side=Left
  P : PMIOPort  Port=2  Side=Left
  T : PMIOPort  Port=3  Side=Left
  BiPIn : PMIOPort  Port=4  Side=Left
  A : PMIOPort  Port=5  Side=Right
  B : PMIOPort  Port=6  Side=Right
  BiPOut : PMIOPort  Port=7  Side=Right
  connections:
  BtoT/LConn2 -- PS Gain1/RConn1 -- BtoARegen/LConn2 -- PtoA/LConn2
  BiPOrifice/LConn2 -- PS Abs/RConn1
  AtoT/LConn2 -- PS Gain1/LConn1 -- PS Abs/LConn1 -- S/RConn1 -- PtoB/LConn2
  BtoARegen/RConn1 -- StickRegenCV/LConn1 -- Volume Regen Valve/LConn1
  T/RConn1 -- BtoT/RConn1 -- AtoT/RConn1
  BiPOrifice/RConn1 -- BiPOut/RConn1
  BiPOrifice/LConn1 -- BiPIn/RConn1
  PtoA/RConn1 -- A/RConn1 -- StickRegenCV/RConn1 -- AtoT/LConn1
  P/RConn1 -- PtoB/LConn1 -- PtoA/LConn1
  BtoARegen/LConn1 -- PtoB/RConn1 -- BtoT/LConn1 -- B/RConn1

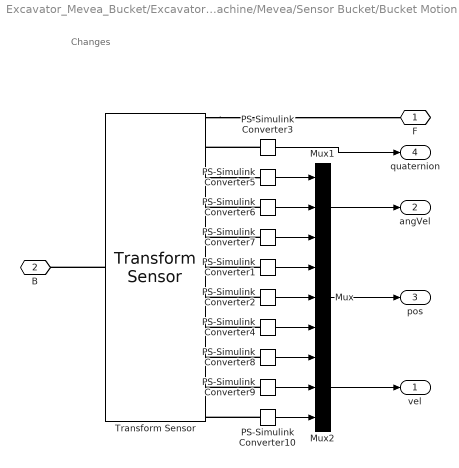
== system Excavator_Mevea_Bucket/Excavator/Machine/Mevea/Sensor Bucket/Bucket Motion Sensor ==
  note: Changes
  Mux : Mux  Inputs=3
  Mux1 : Mux  Inputs=3
  Mux2 : Mux  Inputs=3
  PS-Simulink Converter1 : nesl_utility/PS-Simulink Converter  PhysicalDomain=network_engine_domain  SubClassName=ps_output  LeftPortType=input  RightPortType=output  PseudoPeriodic=off  Frequencies=[]  VectorFormat=inherit  Unit=m  AffineConversion=off
  PS-Simulink Converter10 : nesl_utility/PS-Simulink Converter  PhysicalDomain=network_engine_domain  SubClassName=ps_output  LeftPortType=input  RightPortType=output  PseudoPeriodic=off  Frequencies=[]  VectorFormat=inherit  Unit=m/s  AffineConversion=off
  PS-Simulink Converter2 : nesl_utility/PS-Simulink Converter  PhysicalDomain=network_engine_domain  SubClassName=ps_output  LeftPortType=input  RightPortType=output  PseudoPeriodic=off  Frequencies=[]  VectorFormat=inherit  Unit=m  AffineConversion=off
  PS-Simulink Converter3 : nesl_utility/PS-Simulink Converter  PhysicalDomain=network_engine_domain  SubClassName=ps_output  LeftPortType=input  RightPortType=output  PseudoPeriodic=off  Frequencies=[]  VectorFormat=inherit  Unit=1  AffineConversion=off
  PS-Simulink Converter4 : nesl_utility/PS-Simulink Converter  PhysicalDomain=network_engine_domain  SubClassName=ps_output  LeftPortType=input  RightPortType=output  PseudoPeriodic=off  Frequencies=[]  VectorFormat=inherit  Unit=m  AffineConversion=off
  PS-Simulink Converter5 : nesl_utility/PS-Simulink Converter  PhysicalDomain=network_engine_domain  SubClassName=ps_output  LeftPortType=input  RightPortType=output  PseudoPeriodic=off  Frequencies=[]  VectorFormat=inherit  Unit=deg/s  AffineConversion=off
  PS-Simulink Converter6 : nesl_utility/PS-Simulink Converter  PhysicalDomain=network_engine_domain  SubClassName=ps_output  LeftPortType=input  RightPortType=output  PseudoPeriodic=off  Frequencies=[]  VectorFormat=inherit  Unit=deg/s  AffineConversion=off
  PS-Simulink Converter7 : nesl_utility/PS-Simulink Converter  PhysicalDomain=network_engine_domain  SubClassName=ps_output  LeftPortType=input  RightPortType=output  PseudoPeriodic=off  Frequencies=[]  VectorFormat=inherit  Unit=deg/s  AffineConversion=off
  PS-Simulink Converter8 : nesl_utility/PS-Simulink Converter  PhysicalDomain=network_engine_domain  SubClassName=ps_output  LeftPortType=input  RightPortType=output  PseudoPeriodic=off  Frequencies=[]  VectorFormat=inherit  Unit=m/s  AffineConversion=off
  PS-Simulink Converter9 : nesl_utility/PS-Simulink Converter  PhysicalDomain=network_engine_domain  SubClassName=ps_output  LeftPortType=input  RightPortType=output  PseudoPeriodic=off  Frequencies=[]  VectorFormat=inherit  Unit=m/s  AffineConversion=off
  Transform Sensor : sm_lib/Frames and Transforms/Transform Sensor  MeasurementFrame=Base  RotationSequence=XYZ  SenseAngle=off  SenseAxis=off  SenseQ=on  SenseR=off  SenseRotationSequence=off  SenseOmegaX=on  SenseOmegaY=on  SenseOmegaZ=on  SenseOmega=off  SenseQDot=off  SenseRDot=off  SenseRotationSequenceDot=off  SenseAlphaX=off  SenseAlphaY=off  SenseAlphaZ=off  SenseAlpha=off  SenseQDDot=off  SenseRDDot=off  SenseX=on  SenseY=on  SenseZ=on  SenseXYZ=off  SenseRad=off  SenseAzim=off  SenseDist=off  SenseInc=off  SenseXDot=on  SenseYDot=on  SenseZDot=on  SenseXYZDot=off  SenseRadDot=off  SenseAzimDot=off  SenseDistDot=off  SenseIncDot=off  SenseXDDot=off  SenseYDDot=off  SenseZDDot=off  SenseXYZDDot=off  SenseRadDDot=off  SenseAzimDDot=off  SenseDistDDot=off  SenseIncDDot=off
      settings: AttributesFormatString=Measurement Frame: %<MeasurementFrame>
  F : PMIOPort  Side=Left
  B : PMIOPort  Port=2  Side=Left
  vel : Outport
  angVel : Outport  Port=2
  pos : Outport  Port=3
  quaternion : Outport  Port=4
  wires:
  PS-Simulink Converter4/1 -> Mux/3
  PS-Simulink Converter2/1 -> Mux/2
  PS-Simulink Converter1/1 -> Mux/1
  Mux/1 -> pos/1
  PS-Simulink Converter3/1 -> quaternion/1
  PS-Simulink Converter5/1 -> Mux1/1
  PS-Simulink Converter6/1 -> Mux1/2
  PS-Simulink Converter7/1 -> Mux1/3
  PS-Simulink Converter8/1 -> Mux2/1
  PS-Simulink Converter9/1 -> Mux2/2
  PS-Simulink Converter10/1 -> Mux2/3
  Mux1/1 -> angVel/1
  Mux2/1 -> vel/1
  connections:
  PS-Simulink Converter3/LConn1 -- Transform Sensor/RConn2
  Transform Sensor/LConn1 -- B/RConn1
  Transform Sensor/RConn1 -- F/RConn1
  PS-Simulink Converter10/LConn1 -- Transform Sensor/RConn11
  PS-Simulink Converter9/LConn1 -- Transform Sensor/RConn10
  PS-Simulink Converter8/LConn1 -- Transform Sensor/RConn9
  PS-Simulink Converter4/LConn1 -- Transform Sensor/RConn8
  PS-Simulink Converter2/LConn1 -- Transform Sensor/RConn7
  PS-Simulink Converter1/LConn1 -- Transform Sensor/RConn6
  PS-Simulink Converter7/LConn1 -- Transform Sensor/RConn5
  PS-Simulink Converter6/LConn1 -- Transform Sensor/RConn4
  Transform Sensor/RConn3 -- PS-Simulink Converter5/LConn1

== matlab function Excavator_Mevea_Bucket/Controller/Function Commander/HydraulicCommander ==
  data: swingCmd input; boomCmd input; stickCmd input; bucketCmd input; swingQDmd output; stickHEPr input; stickREPr input; swingSpeed input; boomQDmd output; stickQDmd output; bucketQDmd output; leftPumpDispCmd output; rightPumpDispCmd output; swingMaxQ parameter; boomUpMaxQ parameter; stickOutMaxQ parameter; stickInMaxQ parameter; bucketCloseMaxQ parameter; bucketOpenMaxQ parameter; swingSpoolPos output; boomSpoolPos output; stickSpoolPos output; bucketSpoolPos output; shaftSpeed input; nominalShaftSpeed parameter; minPumpDisp parameter; maxPumpDisp parameter; swingSpeedQGain parameter; swingHighSpeedThreshold parameter
function [swingQDmd, boomQDmd, stickQDmd, bucketQDmd, leftPumpDispCmd, ...
    rightPumpDispCmd, swingSpoolPos, boomSpoolPos, stickSpoolPos, ...
    bucketSpoolPos] = HydraulicCommander( ...
    swingCmd, boomCmd, stickCmd, bucketCmd, stickHEPr, stickREPr, ...
    swingSpeed, swingMaxQ, boomUpMaxQ, stickOutMaxQ, stickInMaxQ, ...
    bucketCloseMaxQ, bucketOpenMaxQ, shaftSpeed, nominalShaftSpeed, ...
    minPumpDisp, maxPumpDisp, swingSpeedQGain, swingHighSpeedThreshold)
%% Initialization
% Flow Rate Demands
swingQDmd = 0; % [lpm]
boomQDmd = 0; % [lpm]
stickQDmd = 0; % [lpm]
bucketQDmd = 0; % [lpm]

% Spool Positions
swingSpoolPos = 0; % [mm]
boomSpoolPos = 0; % [mm]
stickSpoolPos = 0; % [mm]
bucketSpoolPos = 0; % [mm]

% Max Spool Positions
maxPosSpoolPos = 5; % [mm]
maxNegSpoolPos = -5; % [mm]

%% Swing Flow Rate Demand & Spool Position
% Flow Rate
if swingCmd ~= 0
    % Operator command flow rate
    swingOpCmdFlowRate = abs(swingCmd) * swingMaxQ; % [lpm]
  
    % If the swing speed is high or the swing command is opposing the 
    % current speed, use the flow rate directly proportional to the 
    % operator command
    if abs(swingSpeed) > swingHighSpeedThreshold || sign(swingCmd) == sign(swingSpeed)   
        swingQDmd = swingOpCmdFlowRate; % [lpm]
    else
        % Limit the swing flow rate demand based on the current swing speed
        % This limits the flow loss through the swing pressure relief valve
        % during acceleration
        swingSpeedLimitedFlowRate = abs(swingSpeed) * swingSpeedQGain; % [lpm]
        
        % Only use the limited value if it is less than the operator
        % command value
        if swingSpeedLimitedFlowRate < swingOpCmdFlowRate
            swingQDmd = swingSpeedLimitedFlowRate; % [lpm]
        else
            swingQDmd = swingOpCmdFlowRate; % [lpm]
        end
    end 
end

% Spool Position
% Swing Right
if swingCmd > 0
    swingSpoolPos = maxPosSpoolPos; % [mm]
% Swing Left
elseif swingCmd < 0
    swingSpoolPos = maxNegSpoolPos; % [mm]
end

%% Boom Flow Rate Demand & Spool Position
% Boom Up Command Logic - Active Flow
if boomCmd < 0
    boomQDmd = abs(boomCmd) * boomUpMaxQ; % [lpm]
    boomSpoolPos = maxNegSpoolPos; % [mm]
% Boom Down Command Logic - Regenerative Flow
elseif boomCmd > 0
    % For boom down, the valve spool position is varied based on the
    % operator command and there is no pump flow required due to the
    % regenerative flow valve allowing flow from the head end to the rod
    % end during the move. The spool position must be controlled in this 
    % case so that the speed of the boom is proportional to the command. 
    % For boom up, the speed is controlled by limiting the pump flow - but 
    % for boom down, because there is no pump flow, the valve must be used.
    boomSpoolPosFactor = interp1([0 0.10 0.20 0.30 0.40 0.50 0.60 0.70 0.80 0.90 1], ...
                                 [0 0.30 0.45 0.55 0.60 0.70 0.75 0.80 0.85 0.90 1], ...
                                  boomCmd); % [mm]
    boomSpoolPos = maxPosSpoolPos * boomSpoolPosFactor; % [mm]
end

%% Stick Flow Rate Demand & Spool Position
% Stick Out Command Logic - Active Flow
if stickCmd > 0
    stickQDmd = abs(stickCmd) * stickOutMaxQ; % [lpm]
    stickSpoolPos = maxPosSpoolPos; % [mm]
% Stick In Command Logic - Active & Regenerative Flow
elseif stickCmd < 0
    deltaPr = stickREPr - stickHEPr; % [bar]
    if deltaPr > 120
        % When the pressure difference is high, limit the pump flow rate
        % and valve opening to take advantage of the regenerative flow from
        % the rod end. If the valve is opened all the way with a high
        % difference in pressure, the stick velocity will be very high and
        % uncontrolled.  
        stickQDmdFactor = 0.15;
        stickSpoolPosFactor = interp1([0 1], [0 0.55], abs(stickCmd));
    elseif deltaPr > 15
        % When the pressure difference is moderate, start increasing the
        % valve area and pump flow to maintain the velocity.
        stickQDmdFactor = interp1([15 120], [1 0.15], abs(deltaPr));
        stickSpoolPosFactor = interp1([0 1], [0 0.75], abs(stickCmd));
    else
        % When the pressure difference is low, or the head end pressure is
        % higher than the rod end, open the valve completely and allow full
        % pump flow.
        stickQDmdFactor = 1;
        stickSpoolPosFactor = 1;
    end
    % Multiply the maximum flow rate and valve position commands by the
    % factors calculated above to obtain the desired values.
    stickQDmd = abs(stickCmd) * stickInMaxQ * stickQDmdFactor; % [lpm]
    stickSpoolPos = maxNegSpoolPos * stickSpoolPosFactor; % [mm]
end

%% Bucket Flow Rate Demand & Spool Position
% Bucket Open Command Logic - Active Flow
if bucketCmd > 0
    bucketQDmd = abs(bucketCmd) * bucketOpenMaxQ; % [lpm]
    bucketSpoolPos = maxPosSpoolPos; % [mm]
% Bucket Close Command Logic - Active Flow
elseif bucketCmd < 0
    bucketQDmd = abs(bucketCmd) * bucketCloseMaxQ; % [lpm]
    bucketSpoolPos = maxNegSpoolPos; % [mm]
end

%% Pump Distribution
% Max pump flow rate
maxRatedPumpQ = (nominalShaftSpeed * maxPumpDisp)/1000; % [lpm]

% Left Pump: Boom, Stick, Swing
leftPumpQDmd = boomQDmd/2 + stickQDmd/2 + swingQDmd; % [lpm]
% Saturate flow rate demand
if leftPumpQDmd > maxRatedPumpQ
    leftPumpQDmd = maxRatedPumpQ; % [lpm]
end

% Right Pump: Boom, Stick, Bucket
rightPumpQDmd = boomQDmd/2 + stickQDmd/2 + bucketQDmd; % [lpm]
% Saturate flow rate demand
if rightPumpQDmd > maxRatedPumpQ
    rightPumpQDmd = maxRatedPumpQ; % [lpm]
end

%% Left Pump Command
% Convert Flow Rate to Displacement
leftPumpDispCmd = 1000 * (leftPumpQDmd/shaftSpeed); % [cc/rev]
% Saturate displacement command
if leftPumpDispCmd < minPumpDisp
    leftPumpDispCmd = minPumpDisp; % [cc/rev]
elseif leftPumpDispCmd > maxPumpDisp
    leftPumpDispCmd = maxPumpDisp; % [cc/rev]
end

%% Right Pump Command
% Convert Flow Rate to Displacement
rightPumpDispCmd = 1000 * (rightPumpQDmd/shaftSpeed); % [cc/rev]
% Saturate displacement command
if rightPumpDispCmd < minPumpDisp
    rightPumpDispCmd = minPumpDisp; % [cc/rev]
elseif rightPumpDispCmd > maxPumpDisp
    rightPumpDispCmd = maxPumpDisp; % [cc/rev]
end
